simulink library "TimestampChecker"  (R2016b)
settings: Solver=VariableStepAuto  StartTime=0.0  StopTime=10.0  RelTol=1e-3
undefined symbols (not defined in the file): maxNonResponsive
settings Model: Creator=Nathan  LastModifiedBy=march

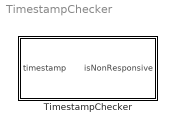
== system TimestampChecker ==
  TimestampChecker : Subsystem

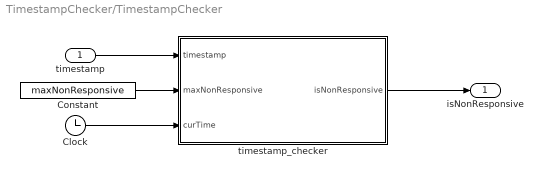
== system TimestampChecker/TimestampChecker ==
  timestamp : Inport
  Clock : Clock
  Constant : Constant  Value=maxNonResponsive  VectorParams1D=off  SampleTime=-1
  timestamp_checker : MATLAB Function  TreatAsAtomicUnit=on
  isNonResponsive : Outport
  wires:
  timestamp_checker/1(isNonResponsive) -> isNonResponsive/1
  timestamp/1 -> timestamp_checker/1(timestamp)
  Constant/1 -> timestamp_checker/2(maxNonResponsive)
  Clock/1 -> timestamp_checker/3(curTime)

== matlab function TimestampChecker/timestamp_checker ==
  data: timestamp input; isNonResponsive output; maxNonResponsive input; curTime input
function isNonResponsive = timestamp_checker(timestamp,maxNonResponsive, curTime)
persistent lastTimestamp;
persistent lastResponseTime;

%Initialize lastTimeStamp and lastResponseTime when model starts
if(isempty(lastTimestamp))
    lastTimestamp = 0;
    lastResponseTime = 0;
end

if((timestamp ~= lastTimestamp))
    lastResponseTime = curTime; % so this stays constant when lastTimeStamp == timestamp
end

if(curTime - lastResponseTime > maxNonResponsive)
    % when there is no response for longer than maxNoResponse, set to true
    isNonResponsive = 1;
else
    isNonResponsive = 0;
end

%always update lastTimeStamp
lastTimestamp = timestamp;
end
